simulink subsystem "DisturbanceGenerator_SubSystem"  (R2020b)
settings: Solver=VariableStepAuto  StartTime=0.0  StopTime=10.0  RelTol=1e-3
undefined symbols (not defined in the file): drv, enable_Disturbance, Ts
settings Model: Creator=umberto  LastModifiedBy=Musta

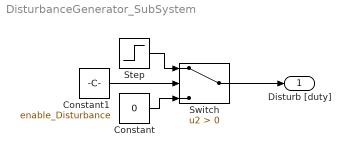
== system DisturbanceGenerator_SubSystem ==
  Constant : Constant  Value=0  SampleTime=Ts
  Constant1 : Constant  Value=enable_Disturbance
  Step : Step  Time=10  After=5/drv.duty2V  SampleTime=Ts
  Switch : Switch  Criteria=u2 > Threshold
  Disturb [duty] : Outport
  wires:
  Constant/1 -> Switch/3
  Step/1 -> Switch/1
  Switch/1 -> Disturb [duty]/1
  Constant1/1 -> Switch/2
